simulink model "DC_Servo"  (R2013a)
settings: Solver=ode45  StartTime=0.0  StopTime=10.0  RelTol=1e-3
undefined symbols (not defined in the file): b, j, kb, kt, L, R
settings Model: Creator=Ahmed  LastModifiedBy=Ahmed

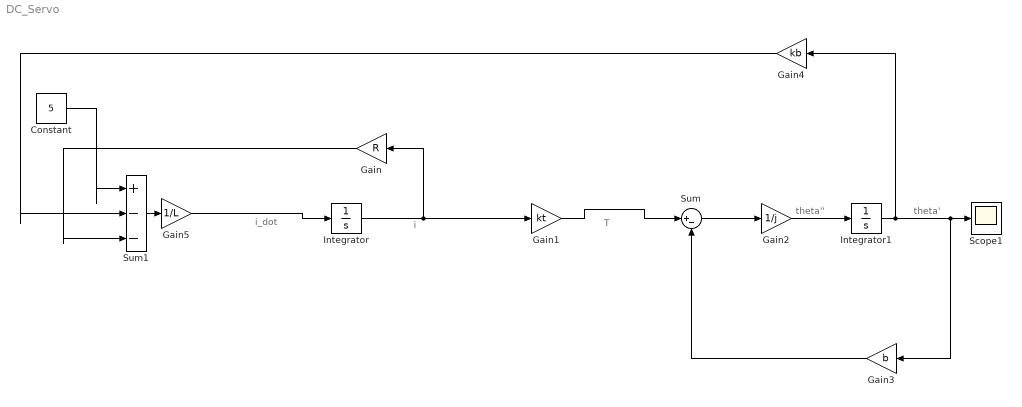
== system DC_Servo ==
  note: theta'
  note: theta''
  note: T
  note: i
  note: i_dot
  Constant : Constant  Value=5
  Gain : Gain  Gain=R
  Gain1 : Gain  Gain=kt
  Gain2 : Gain  Gain=1/j
  Gain3 : Gain  Gain=b
  Gain4 : Gain  Gain=kb
  Gain5 : Gain  Gain=1/L
  Integrator : Integrator
  Integrator1 : Integrator
  Scope1 : Scope
  Sum : Sum  Inputs=|+-
  Sum1 : Sum  Inputs=|+--
  wires:
  Integrator/1 -> Gain1/1, Gain/1
  Gain5/1 -> Integrator/1
  Gain1/1 -> Sum/1
  Sum/1 -> Gain2/1
  Gain2/1 -> Integrator1/1
  Integrator1/1 -> Gain4/1, Gain3/1, Scope1/1
  Gain3/1 -> Sum/2
  Constant/1 -> Sum1/1
  Gain4/1 -> Sum1/2
  Gain/1 -> Sum1/3
  Sum1/1 -> Gain5/1
